simulink model "EOM_6DOF"  (R2023b)
settings: Solver=VariableStepAuto  StartTime=0.0  StopTime=30  RelTol=1e-3
libraries: shared6dof x1
settings Model: Creator=kay18  LastModifiedBy=kay18
settings OptimizationCC: BlockReduction=off  DefaultParameterBehavior=Inlined  BufferReuse=off

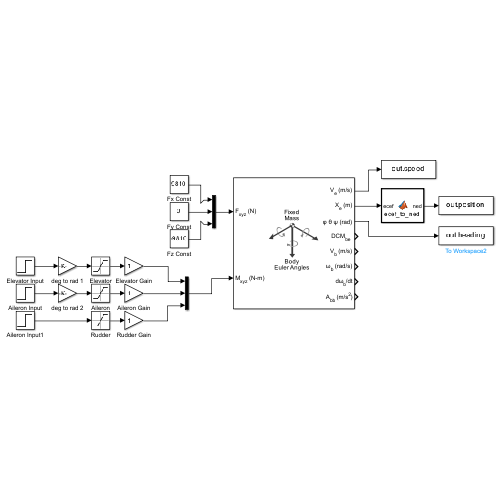
[thumbnail: Simulink's stored preview of the top-level diagram]
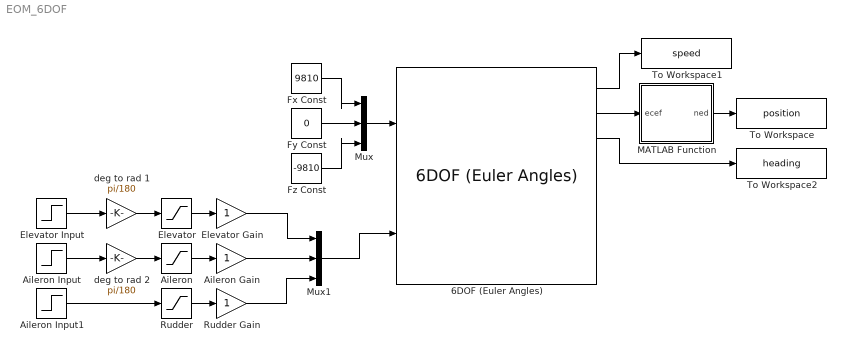
== system EOM_6DOF ==
  6DOF (Euler Angles) : shared6dof/6DOF (Euler Angles)  units=Metric (MKS)  mtype=Fixed  rep=Euler Angles  xme_0=[-2706176.8; -4261051.6; 3885743.7]  Vm_0=[60,0,0]  eul_0=[0 0 0]  pm_0=[0 0 0]  mass_0=1088.62  mass_e=0.5  mass_f=2.0  inertia=[948 0 0; 0 1346 0; 0 0 1967]  inertia_e=eye(3)  inertia_f=2*eye(3)  k_quat=1.0  vre_flag=on  abi_flag=off  aMode=0  xme_statename=''  Vm_statename=''  eul_statename=''  quat_statename=''  pm_statename=''  mass_statename=''
  Aileron : Saturate
  Aileron Gain : Gain
  Aileron Input : Step  After=5  SampleTime=0
  Aileron Input1 : Step  After=5  SampleTime=0
  Elevator : Saturate
  Elevator Gain : Gain
  Elevator Input : Step  After=5  SampleTime=0
  Fx Const : Constant  Value=9810
  Fy Const : Constant  Value=0
  Fz Const : Constant  Value=-9810
  MATLAB Function : MATLAB Function  TreatAsAtomicUnit=on
  Mux : Mux  Inputs=3
  Mux1 : Mux  Inputs=3
  Rudder : Saturate
  Rudder Gain : Gain
  To Workspace : ToWorkspace  VariableName=position  SampleTime=-1
  To Workspace1 : ToWorkspace  VariableName=speed  SampleTime=-1
  To Workspace2 : ToWorkspace  VariableName=heading  SampleTime=-1
  deg to rad 1 : Gain  Gain=pi/180
  deg to rad 2 : Gain  Gain=pi/180
  wires:
  Mux/1 -> 6DOF (Euler Angles)/1
  Mux1/1 -> 6DOF (Euler Angles)/2
  Fx Const/1 -> Mux/1
  Fy Const/1 -> Mux/2
  Fz Const/1 -> Mux/3
  Rudder/1 -> Rudder Gain/1
  Aileron/1 -> Aileron Gain/1
  Elevator/1 -> Elevator Gain/1
  Elevator Gain/1 -> Mux1/1
  Aileron Gain/1 -> Mux1/2
  Rudder Gain/1 -> Mux1/3
  deg to rad 1/1 -> Elevator/1
  deg to rad 2/1 -> Aileron/1
  Aileron Input1/1 -> Rudder/1
  Elevator Input/1 -> deg to rad 1/1
  Aileron Input/1 -> deg to rad 2/1
  6DOF (Euler Angles)/2 -> MATLAB Function/1(ecef)
  MATLAB Function/1(ned) -> To Workspace/1
  6DOF (Euler Angles)/1 -> To Workspace1/1
  6DOF (Euler Angles)/3 -> To Workspace2/1

== matlab function EOM_6DOF/MATLAB Function ==
  data: ned output; ecef input double size=[1 3]
function ned = ecef_to_ned(ecef)
    % Reference position in LLA
    lat0 = 37.7749; lon0 = -122.4194; alt0 = 1000;

    % Convert reference to ECEF
    ecef_ref = lla2ecef_custom([lat0, lon0, alt0]);

    % Delta vector
    delta = ecef - ecef_ref;

    % Convert to radians
    lat0 = deg2rad(lat0);
    lon0 = deg2rad(lon0);

    % Rotation matrix ECEF->NED
    R = [ -sin(lat0)*cos(lon0), -sin(lat0)*sin(lon0),  cos(lat0);
          -sin(lon0),           cos(lon0),           0;
          -cos(lat0)*cos(lon0), -cos(lat0)*sin(lon0), -sin(lat0)];

    % Compute NED
    ned_col = R * delta';
    ned = ned_col';

end

function ecef = lla2ecef_custom(lla)
    lat = deg2rad(lla(1));
    lon = deg2rad(lla(2));
    alt = lla(3);

    a = 6378137.0;
    f = 1/298.257223563;
    e2 = 2*f - f^2;

    N = a / sqrt(1 - e2 * sin(lat)^2);

    Xe = (N + alt) * cos(lat) * cos(lon);
    Ye = (N + alt) * cos(lat) * sin(lon);
    Ze = (N * (1 - e2) + alt) * sin(lat);

    ecef = [Xe, Ye, Ze];
end
